simulink model "xpctank1"  (Simulink 8.0)
settings: Solver=ode4  StartTime=0.0  StopTime=99999  FixedStep=0.001  RelTol=1e-3
libraries: xpclib x2
settings Model: Creator=mvetsch  LastModifiedBy=desheng  SimulationMode=external  BufferReuse=off
settings SolverCC: AutoInsertRateTranBlk=on
settings DataIOCC: LimitDataPoints=off  SignalLoggingSaveFormat=ModelDataLogs  SignalLoggingName=logsOut
settings OptimizationCC: BlockReduction=off  BooleanDataType=off  InlineInvariantSignals=on  OptimizeBlockIOStorage=off  BufferReuse=off  ExpressionFolding=off  LocalBlockOutputs=off  InitFltsAndDblsToZero=on
settings DebuggingCC: SaveWithParameterizedLinksMsg=none  CheckExecutionContextPreStartOutputMsg=on  CheckExecutionContextRuntimeOutputMsg=on  SignalResolutionControl=TryResolveAllWithWarning  SolverPrmCheckMsg=none  MultiTaskDSMMsg=warning  MultiTaskCondExecSysMsg=none  StrictBusMsg=None
settings HardwareCC: ProdIntDivRoundTo=Zero  ProdEndianess=LittleEndian  ProdHWDeviceType=Generic->32-bit x86 compatible
settings RTWCC: SystemTargetFile=xpctarget.tlc  TemplateMakefile=xpc_default_tmf  Description=xPC Target  ProcessScript=xpctarget_make_rtw_hook  IncludeERTFirstTime=on  RTWCompilerOptimization=On
settings xpcTargetCC: TargetFcnLib=ansi_tfl_tmw.mat  CodeReplacementLibrary=XPC_BLAS  ParMdlRefBuildCompliant=on  ConcurrentExecutionCompliant=on  CombineSignalStateStructs=off  GRTInterface=on  xPCTaskExecutionProfile=off  xPCRL32EventNumber=5000  xpcObjCom=on  xPCLoadParamSetFile=off  xPCConcurrentTasks=off  xPCEnableSFAnimation=off

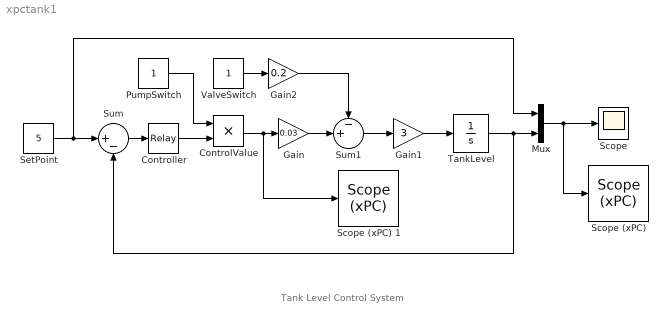
== system xpctank1 ==
  note: Tank Level Control System
  ControlValue : Product  Description=ToxPC(1,2,3)=OnSwitchValue OffSwitchValue OnOutputValue;  SaturateOnIntegerOverflow=on  RndMeth=Zero  InputSameDT=on  OutDataTypeStr=Inherit: Same as first input
  Controller : Relay  Description=xPCTag(1,2,3)=ToOnSwitch ToOffSwitch ToOnOutput;  OnSwitchValue=1  OffSwitchValue=-1  OnOutputValue=10
  Gain : Gain  Gain=0.03  SaturateOnIntegerOverflow=on  OutDataTypeStr=Inherit: Same as input  ParamDataTypeStr=Inherit: Same as input
  Gain1 : Gain  Gain=3  SaturateOnIntegerOverflow=on  OutDataTypeStr=Inherit: Same as input  ParamDataTypeStr=Inherit: Same as input
  Gain2 : Gain  Gain=0.2  SaturateOnIntegerOverflow=on  OutDataTypeStr=Inherit: Same as input  ParamDataTypeStr=Inherit: Same as input
  Mux : Mux  Inputs=2
  PumpSwitch : Constant  Description=xPCTag(1)=ToPumpSwitch;
  Scope : Scope
      settings: YMin=0  YMax=15
  "Scope (xPC) " : xpclib/Misc./Scope (xPC)   scopeno=1  scopetype=Target  autostart=on  viewmode=Graphical rolling  formatstr='%15.6f'  grid=on  ylimits=[0,10]  nosamples=500  noprepostsamples=0  interleave=100  triggermode=FreeRun  triggersignal=1  triggerlevel=0.0  triggerslope=Either  triggerscope=1  triggersample=0  filename=data.dat  mode=Lazy  writesize=512  autorestart=off  dynamicfilemode=off  maxwritefilesize=512*1024^2
  Scope (xPC) 1 : xpclib/Misc./Scope (xPC)   scopeno=2  scopetype=Target  autostart=on  viewmode=Graphical rolling  formatstr='%15.6f'  grid=on  ylimits=[0,15]  nosamples=500  noprepostsamples=0  interleave=100  triggermode=FreeRun  triggersignal=1  triggerlevel=0.0  triggerslope=Either  triggerscope=1  triggersample=0  filename=data.dat  mode=Lazy  writesize=512  autorestart=off  dynamicfilemode=off  maxwritefilesize=512*1024^2
  SetPoint : Constant  Description=xPCTag(1)=ToSetPoint;  Value=5
  Sum : Sum  Inputs=|+-  SaturateOnIntegerOverflow=on  InputSameDT=on  OutDataTypeStr=Inherit: Same as first input
  Sum1 : Sum  Inputs=-+|  SaturateOnIntegerOverflow=on  InputSameDT=on  OutDataTypeStr=Inherit: Same as first input
  TankLevel : Integrator  LimitOutput=on  UpperSaturationLimit=+inf  LowerSaturationLimit=0
  ValveSwitch : Constant  Description=xPCTag(1)=ToValueSwitch;
  wires:
  Sum/1 -> Controller/1
  PumpSwitch/1 -> ControlValue/1
  Gain/1 -> Sum1/2
  Sum1/1 -> Gain1/1
  Gain1/1 -> TankLevel/1
  Gain2/1 -> Sum1/1
  ValveSwitch/1 -> Gain2/1
  SetPoint/1 -> Sum/1, Mux/1
  Mux/1 -> Scope/1, "Scope (xPC) "/1
  Controller/1 -> ControlValue/2
  ControlValue/1 -> Gain/1, Scope (xPC) 1/1
  TankLevel/1 -> Mux/2, Sum/2
